simulink library "canBswLib"  (R2023b)
settings: Solver=VariableStepAuto  StartTime=0.0  StopTime=10.0  RelTol=1e-3
undefined symbols (not defined in the file): Data, Extended, ID, Length
libraries: can_bswapi x15, simulink x12, hdlsllib x5, $bdroot x4, dspswit3 x2, bamFsm x1
settings Model: Creator=zon07  LastModifiedBy=Professional
settings SFSimCC: SimTargetLang=C++

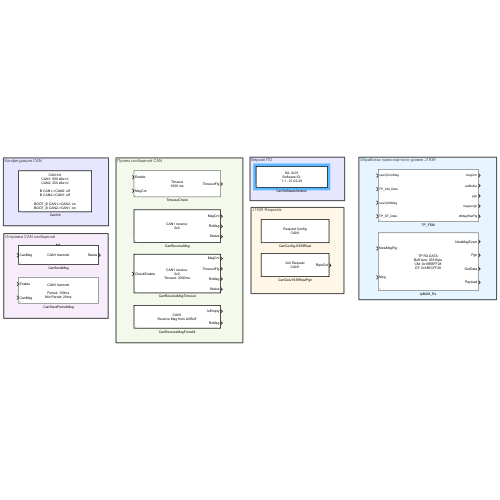
[thumbnail: Simulink's stored preview of the top-level diagram]
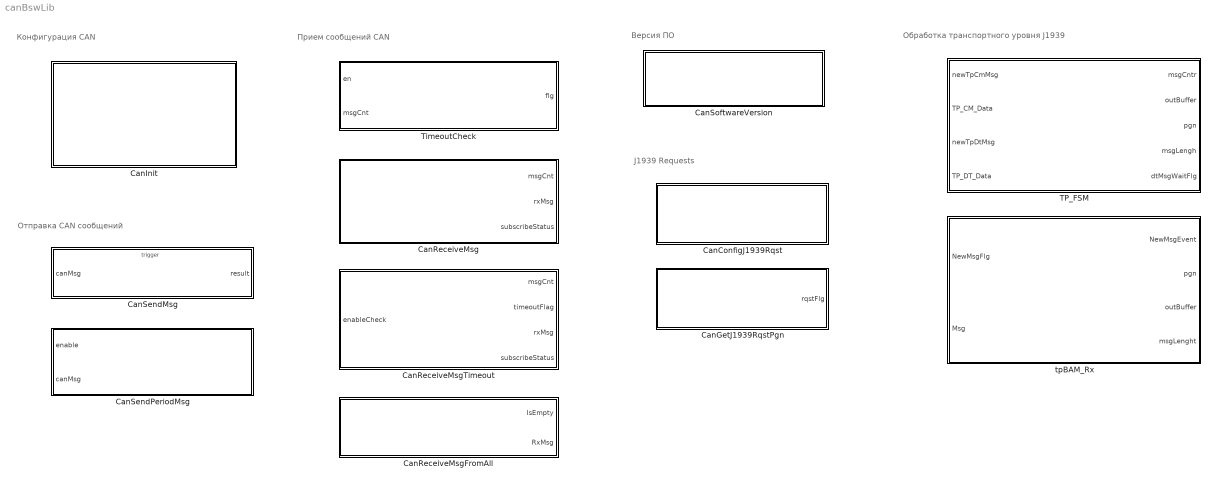
== system canBswLib ==
  note: Обработка транспортного уровня J1939
  note: Версия ПО
  note: J1939 Requests
  note: Отправка CAN сообщений
  note: Конфигурация CAN
  note: Прием сообщений CAN
  CanConfigJ1939Rqst : Subsystem  TreatAsAtomicUnit=on  mask(Request Config){can='CAN1', id=0x18EA3128, onlyPgnFlg=on, fromAllFlg=on}
      mask prompts: can "CAN Number"; id "Rqst Id:"; onlyPgnFlg "Принимать только по PGN"; fromAllFlg "Принимать запрос "Для всех""
      mask help:
      | Данный блок устанавливает с какого ID будут приниматься запросы.
      | CAN Number: номер CAN;
      | Rqst Id: Id запроса;
      | Флаг "Флаг принимать только по PGN" - SA источника запроса будет игнорироваться;
      | Флаг "Принимать запрос "Для всех" - Пример если установлен 0x18EA3128, так же будет обрабатываться 0x18EAFF28;
      mask init:
      | block_name = "Request Config\n" + "CAN" + num2str(can);
      mask TypeOptions can: 'CAN1' | 'CAN2'
      mask DialogControl ParameterGroupVar Prompt: CAN:
      mask DialogControl Container3 Prompt: Parameters
      mask Display: disp(block_name);
  CanGetJ1939RqstPgn : Subsystem  TreatAsAtomicUnit=on  mask(Get request for PGN){can='CAN1', pgn=0x0000}
      mask prompts: can "CAN Number"
      mask help:
      | Функция возвращает true на один шаг,если был получен запрос на утсановленный PGN.
      | Максимум 16 уникальных Pgn.
      mask init:
      | block_name = "0x" + dec2hex(pgn) + " Request\n" + "CAN" + num2str(can);
      mask TypeOptions can: 'CAN1' | 'CAN2'
      mask DialogControl ParameterGroupVar Prompt: CAN
      mask Display:
      | disp(block_name)
      | port_label('output', 1, 'RqstСnt');
  CanSoftwareVersion : Subsystem  LoadFcn=|  TreatAsAtomicUnit=on  mask(Software Version CAN){software_version=0, model_number=1, version=1, subversion=1, firmware_date="21.02.25", date_update=on, sa=0x31, id=0x18EAFF28, id_1=0x18EAFF28}
      | null_str = """00.00.00""";
      | read_str = get_param(gcb, 'firmware_date');
      | 
      | if (read_str == null_str)
      |     write_str = """" + string(datetime('now', 'Format', 'dd.MM.yy')) + """";
      |     set_param(gcb, 'firmware_date', write_str);
      | end
      | 
      | update = get_param(gcb, 'date_update');
      | 
      | switch (update)
      |     case 'on'
      |         write_str = """" + string(datetime('now', 'Format', 'dd.MM.yy')) + """";
      |         set_param(gcb, 'firmware_date', write_str);
      |     case 'off'
      |         %Nothing to do
      | end
      | 
      | clear null_str read_str write_str update;
      mask prompts: software_version "Software version"; model_number "Model number:"; version "Firmware version:"; subversion "Firmware subversion:"; firmware_date "Date:"; date_update "Update on model startup"; id "Message ID:"; id_1 "Message ID:"
      mask help: Процесс приема запроса и отправки версии ПО в CAN согласно J1939.
      mask init:
      | software_version = char(3) + "-" + num2str(model_number, '%02.0f') + "*" + num2str(version, '%02.0f') + "." + num2str(subversion) + "*" + firmware_date + "*";
      | block_name = "SA: 0x" + num2str(dec2hex(sa)) + "\nSoftware ID:\n" + num2str(version) + "." + num2str(subversion) + " - " + firmware_date;
      settings: CopyFcn=|
      | null_str = """00.00.00""";
      | read_str = get_param(gcb, 'firmware_date');
      | 
      | if (read_str == null_str)
      |     write_str = """" + string(datetime('now', 'Format', 'dd.MM.yy')) + """";
      |     set_param(gcb, 'firmware_date', write_str);
      | end
      | 
      | clear null_str read_str write_str;
      settings: MoveFcn=|
      | null_str = """00.00.00""";
      | read_str = get_param(gcb, 'firmware_date');
      | 
      | if (read_str == null_str)
      |     write_str = """" + string(datetime('now', 'Format', 'dd.MM.yy')) + """";
      |     set_param(gcb, 'firmware_date', write_str);
      | end
      | 
      | clear null_str read_str write_str;
      mask TypeOptions id: СanReceiveMsg/id
      mask TypeOptions id_1: СanReceiveMsg1/id
      mask DialogControl ParameterGroupVar Prompt: Firmware version
      mask DialogControl Container3 Prompt: Date
      mask DialogControl Container6 Prompt: CAN SA
      mask DialogControl Container4 Prompt: CAN1 Request
      mask DialogControl Container5 Prompt: CAN2 Request
      mask Display: disp(block_name);
  TP_FSM : Subsystem  mask(J1939 TP Msg Rx Fsm){buffSize=255}
      mask prompts: buffSize "Размер буффера, байт:"
      mask help: Машина состояний приема сообщений по Transport Protocol J1939
  TimeoutCheck : Subsystem  mask(Check TimeOut){timeout_ms=1000}
      mask prompts: timeout_ms "Timeout, ms"
      mask help: Проверка таймаута для CAN сообщений
      mask init:
      | block_name = "Timeout\n" + num2str(timeout_ms) + " ms";
      mask DialogControl ParameterGroupVar Prompt: Параметры
      mask Display:
      | disp(block_name);
      | port_label('input', 1, 'Enable');
      | port_label('input', 2, 'MsgCnt');
      | port_label('output', 1, 'TimeoutFlg');
  tpBAM_Rx : Subsystem  mask(TP RX DATA){tpCmId=0x18EBFF28, tpDtId=0x18ECFF28, buffSize=255}
      mask prompts: tpCmId "CAN ID TP.CM:"; tpDtId "CAN ID DT.CM:"; buffSize "Размер буффера, байт:"
      mask help:
      | Прием сообщений по транспортному протоколу J1939.
      | Порты:
      | 1) NewMsgEvent - событие(вызов) при получении(сборке) нового сообщения;
      | 2) Pgn - PGN принятого сообщений;
      | 3) OutData - массив данных собранного сообщений (длина равна BuffSize заданного в настройках);
      | 4) MsgLenght - длина полезных данных в буффере;
      | 5) DtMsgWaitFlg - флаг ожидания приема сообщения данных TP.DT;
      |
      | !!! При неудачном приеме - буффер очищается (0xFF).
      mask init:
      | blockName = "TP RX DATA\n" + "Buff size: " + num2str(buffSize) + " Byte"...
      |                 + "\nCM: 0x" + dec2hex(tpCmId)...
      |                 + "\nDT: 0x" + dec2hex(tpDtId);
      mask TypeOptions buffSize: TP_FSM/buffSize
      mask DialogControl ParameterGroupVar Prompt: Параметры
      mask Display:
      | disp(blockName);
      | port_label('input', 1, 'NewMsgFlg');
      | port_label('input', 2, 'Msg');
      | 
      | port_label('output', 1, 'NewMsgEvent');
      | port_label('output', 3, 'OutData');
      | port_label('output', 2, 'Pgn');
      | port_label('output', 4, 'Payload');
  СanInit : Subsystem  TreatAsAtomicUnit=on  mask(Инициализация CAN){bitrate_can_1=500 кбит/с, brigdeCan1to2Flg=off, bootBrigdeCan1to2Flg=on, bitrate_can_2=250 кбит/с, brigdeCan2to1Flg=off, bootBrigdeCan2to1Flg=on}
      mask prompts: bitrate_can_1 "Скорость шины CAN 1"; brigdeCan1to2Flg "Проброс сообщений из CAN1 в CAN2"; bootBrigdeCan1to2Flg "Проброс сообщений бутлоадера из CAN1 в CAN2"; bitrate_can_2 "Скорость шины CAN 2"; brigdeCan2to1Flg "Проброс сообщений из CAN2 в CAN1"; bootBrigdeCan2to1Flg "Проброс сообщений бутлоадера из CAN2 в CAN1"
      mask help:
      | Выбор скорости передачи данных для CAN1 и CAN2;
      | Выбор необходимости Bridge-режима (проброса) для каждого CAN;
      | BOOT_RS_ID - CAN_ID по которому будет происходить сброс контроллера (возможно уберем в будущем).
      mask init:
      | maskObj = Simulink.Mask.get(gcb);
      | speedCan1 = maskObj.getParameter('bitrate_can_1').Value;
      | speedCan2 = maskObj.getParameter('bitrate_can_2').Value;
      | 
      | bridge1_2 = maskObj.getParameter('brigdeCan1to2Flg').Value;
      | bridge2_1 = maskObj.getParameter('brigdeCan2to1Flg').Value;
      | 
      | bootBrigde1_2 = maskObj.getParameter('bootBrigdeCan1to2Flg').Value;
      | bootBrigde2_1 = maskObj.getParameter('bootBrigdeCan2to1Flg').Value;
      | 
      | block_name = "CAN Init" + "\n" + "CAN1: " + speedCan1...
      |                         + "\n" + "CAN2: " + speedCan2...
      |                         + "\n\n" + "B CAN1->CAN2: " + bridge1_2...
      |                         + "\n" + "B CAN2->CAN1: " + bridge2_1...
      |                         + "\n\n" + "BOOT_B CAN1->CAN2: " + bootBrigde1_2...
      |                         + "\n" + "BOOT_B CAN2->CAN1: " + bootBrigde2_1;
      mask TypeOptions bitrate_can_1: 125 кбит/с | 250 кбит/с | 500 кбит/с | 1000 кбит/с
      mask TypeOptions bitrate_can_2: 125 кбит/с | 250 кбит/с | 500 кбит/с | 1000 кбит/с
      mask DialogControl Container Prompt: CAN1
      mask DialogControl Container1 Prompt: CAN2
      mask Display: disp(block_name);
  СanReceiveMsg : Subsystem  TreatAsAtomicUnit=on  mask(Прием Can-сообщения по "подписке"){can=CAN1, id=0x0, sample_time=-1}
      mask prompts: id "Message ID:"; sample_time "Sample time:"
      mask help:
      | Задайте идентификатор сообщения CAN которое необходимо получать.
      |
      | На выходе rxMsg данные будут в виде BUS:CAN_MESSAGE_BUS
      | На выходе msgCnt будет счетчик количества принятых собщений uint32.
      |
      | Ограничение на количество блоков с уникальным ID - 128 блока (с учетом СanReceiveMsgTimeout) для кажого модуля CAN.
      | Если количество ID превышено и подписка не удалась, на выходе Status будет значение False (0) ;
      |
      | Sample time - период выполнения блока. Должен быть больше шага моделирования. Значение -1 задаёт Sample time как наследуемый.
      mask init:
      | block_name = "CAN" + num2str(can) + " receive:\n0x" + dec2hex(id);
      mask TypeOptions can: CAN1 | CAN2
      mask DialogControl ParameterGroupVar Prompt: Параметры
      mask Display:
      | disp(block_name);
      | port_label('output', 1, 'MsgCnt');
      | port_label('output', 2, 'RxMsg');
      | port_label('output', 3, 'Status');
  СanReceiveMsgFromAll : Subsystem  TreatAsAtomicUnit=on  mask(Получить сообщений из кольцевого буффера CAN){can=CAN1}
      mask help:
      | Получение сообщения из кольцевого буффера CAN.
      | IsEmpty - Флаг сигнализирующий, что буффер пуст.
      |
      | Одиночный вызов - считает одно сообщение из буффера.
      | Данный блок целесообразно использовать в конструкции с циклом while.
      | Так можно считывать все сообщения(и повторяющиеся ID) принятые за шаг выполнения.
      mask init:
      | block_name = "CAN" + num2str(can) + "\nReceive Msg from All Buff";
      mask TypeOptions can: CAN1 | CAN2
      mask DialogControl ParameterGroupVar Prompt: Параметры
      mask Display:
      | disp(block_name);
      | port_label('output', 1, 'IsEmpty');
      | port_label('output', 2, 'RxMsg');
  СanReceiveMsgTimeout : Subsystem  TreatAsAtomicUnit=on  mask(Can Message Rx){id=0, can='CAN1', timeout_ms=2000, sample_time=-1}
      mask prompts: timeout_ms "Timeout, ms"; sample_time "Sample time, s:"
      mask help:
      | Задайте идентификатор сообщения CAN которое необходимо получать.
      |
      | На выходе rxMsg данные будут в виде BUS:CAN_MESSAGE_BUS
      | На выходе msgCnt будет счетчик количества принятых собщений uint32.
      |
      | Ограничение на количество блоков с уникальным ID - 128 блока(с учетом СanReceiveMsg)для кажого модуля CAN.
      | Если количество ID превышено и подписка не удалась, на выходе Status будет значение False (0) ;
      |
      | Sample time - период выполнения блока. Должен быть больше шага моделирования. Значение -1 задаёт Sample time как наследуемый.
      |
      | enableCheck - включение контроля таймаута;
      | timeoutFlg - флаг контроля таймаута сообщения;
      mask init:
      | block_name = "CAN" + num2str(can) + " receive:\n0x" + dec2hex(id) + "\nTimeout: " + timeout_ms + "ms";
      mask TypeOptions can: 'CAN1' | 'CAN2'
      mask DialogControl Container2 Prompt: Параметры
      mask Display:
      | disp(block_name);
      | port_label('output', 1, 'MsgCnt');
      | port_label('output', 2, 'TimeoutFlg');
      | port_label('output', 3, 'RxMsg');
      | port_label('output', 4, 'Status');
      | port_label('input', 1, 'CheckEnable');
  СanSendMsg : Subsystem  mask(Отправка сообщения CAN){can=CAN1}
      mask help:
      | Выберите CAN шину для передачи сообщения.
      |
      | Порт canMsg - Сообщение для отправки типа Bus: CAN_MESSAGE_BUS.
      |
      | Данный блок, при вызове, поместит сообщений в очередь CAN для отправки.
      |
      | Status - статус выполнения функции (Тип Enum: Statuses)
      mask init:
      | blockName = "CAN" + num2str(can) + " transmit";
      mask TypeOptions can: CAN1 | CAN2
      mask DialogControl ParameterGroupVar Prompt: Параметры
      mask Display:
      | disp(blockName);
      | port_label('input', 1, 'CanMsg');
      | port_label('output', 1, 'Status');
  СanSendPeriodMsg : Subsystem  mask(CanSend){by_period=on, by_dataChange=off, can=CAN1, period_time=0.1, sample_time=0.02}
      mask prompts: by_period "Периодическая отправка"; by_dataChange "По изменению данных"; period_time "Период , сек:"; sample_time "Минимальный период, сек:"
      mask help: Выберите CAN шину для передачи сообщения.<br>Sample time - период выполнения блока. Должен быть больше шага моделирования. Значение -1 задаёт Sample time как наследуемый.<br><br>-Порт enable - включения/выключения отправки.<br>-Порт canMsg - Сообщение для отправки типа Bus: CAN_MESSAGE_BUS(можно создать коммандой canMessageBusType, скопировать и поместить в словарь модели)
      mask init:
      | block_name = "CAN" + num2str(can) + " transmit";
      | period = num2str(period_time * 1000)+ "ms";
      | 
      | if(sample_time == -1)
      |     min_period = "Inherit";
      | else
      |     min_period = num2str(sample_time * 1000)+ "ms";  
      | end
      | 
      | if(by_period == true && by_dataChange == false)
      |     block_name = "CAN" + num2str(can) + " transmit\n\n" + "Period: " + period + "\nMin Period: " + min_period;
      | elseif(by_period == true && by_dataChange == true)
      |     block_name = "CAN" + num2str(can) + " transmit\n\n" + "By Data Change\n" + "Period: " + period + "\nMin Period: " + min_period;
      | elseif(by_period == false && by_dataChange == true)
      |     block_name = "CAN" + num2str(can) + " transmit\n\n" + "By Data Change" + "\nMin Period: " + min_period;
      | else
      |     block_name = "CAN" + num2str(can) + " transmit OFF";
      | end
      mask TypeOptions can: CAN1 | CAN2
      mask DialogControl Container4 Prompt: Настройки:
      mask DialogControl ParameterGroupVar Prompt: Параметры
      mask DialogControl Container3 Prompt: Периоды
      mask Display:
      | disp(block_name);
      | port_label('input', 1, 'Enable');
      | port_label('input', 2, 'CanMsg');

== system canBswLib/CanConfigJ1939Rqst ==
  Constant1 : Constant  Value=0
  Initialize Function : Subsystem  TreatAsAtomicUnit=on
  Terminator : Terminator
  wires:
  Constant1/1 -> Terminator/1

== system canBswLib/CanGetJ1939RqstPgn ==
  Constant : Constant  Value=pgn  OutDataTypeStr=uint32
  Initialize Function : Subsystem  TreatAsAtomicUnit=on
  can : Constant  Value=(can - 1)  OutDataTypeStr=int32
  canApi_getRqstJ1939 : can_bswapi/canApi_getRqstJ1939  SampleTime=-1
  rqstFlg : Outport  OutDataTypeStr=uint32
  wires:
  Constant/1 -> canApi_getRqstJ1939/2
  canApi_getRqstJ1939/1 -> rqstFlg/1
  can/1 -> canApi_getRqstJ1939/1

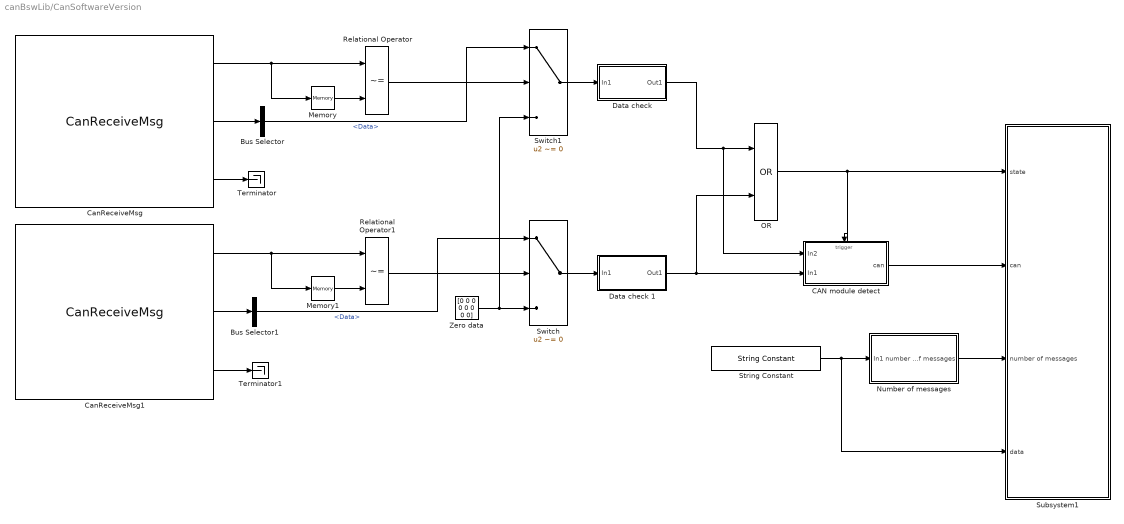
== system canBswLib/CanSoftwareVersion ==
  Bus Selector : BusSelector  OutputSignals=Data
  Bus Selector1 : BusSelector  OutputSignals=Data
  CAN module detect : Subsystem  TreatAsAtomicUnit=on
  Data check : Subsystem
  Data check 1 : Subsystem
  Memory : Memory
  Memory1 : Memory
  Number of messages : Subsystem
  OR : Logic  Operator=OR  AllPortsSameDT=off  OutDataTypeStr=boolean
  Relational Operator : RelationalOperator  Operator=~=  OutDataTypeStr=boolean  RndMeth=Simplest  InputSameDT=off
  Relational Operator1 : RelationalOperator  Operator=~=  OutDataTypeStr=boolean  RndMeth=Simplest  InputSameDT=off
  String Constant : StringConstant  String=software_version
  Subsystem1 : Subsystem
  Switch : Switch  Criteria=u2 ~= 0  RndMeth=Simplest  SaturateOnIntegerOverflow=off  InputSameDT=off
  Switch1 : Switch  Criteria=u2 ~= 0  RndMeth=Simplest  SaturateOnIntegerOverflow=off  InputSameDT=off
  Terminator : Terminator
  Terminator1 : Terminator
  Zero data : Constant  Value=[0 0 0 0 0 0 0 0]  OutDataTypeStr=uint8
  СanReceiveMsg : $bdroot/СanReceiveMsg  can=CAN1  id=id  sample_time=0.2
  СanReceiveMsg1 : $bdroot/СanReceiveMsg  can=CAN2  id=id_1  sample_time=0.2
  wires:
  СanReceiveMsg/3 -> Terminator/1
  СanReceiveMsg1/3 -> Terminator1/1
  Bus Selector1/1 -> Switch/1  "<Data>"
  Relational Operator1/1 -> Switch/2
  Memory1/1 -> Relational Operator1/2
  СanReceiveMsg1/1 -> Relational Operator1/1, Memory1/1
  СanReceiveMsg1/2 -> Bus Selector1/1
  Bus Selector/1 -> Switch1/1  "<Data>"
  СanReceiveMsg/2 -> Bus Selector/1
  Relational Operator/1 -> Switch1/2
  СanReceiveMsg/1 -> Relational Operator/1, Memory/1
  Memory/1 -> Relational Operator/2
  CAN module detect/1(can) -> Subsystem1/2(can)
  OR/1 -> Subsystem1/1(state), CAN module detect/Trigger
  Data check 1/1(Out1) -> CAN module detect/2(In1), OR/2
  Data check/1(Out1) -> CAN module detect/1(In2), OR/1
  Switch/1 -> Data check 1/1(In1)
  Switch1/1 -> Data check/1(In1)
  Zero data/1 -> Switch/3, Switch1/3
  String Constant/1 -> Number of messages/1(In1), Subsystem1/4(data)
  Number of messages/1(number of messages) -> Subsystem1/3(number of messages)

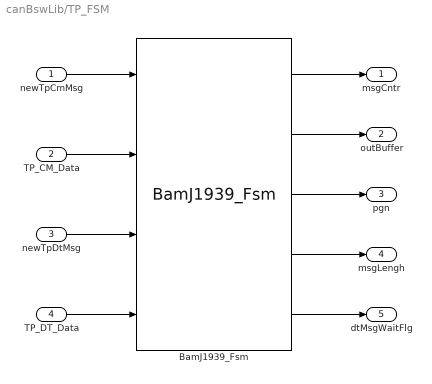
== system canBswLib/TP_FSM ==
  newTpCmMsg : Inport
  TP_CM_Data : Inport  Port=2
  newTpDtMsg : Inport  Port=3
  TP_DT_Data : Inport  Port=4
  BamJ1939_Fsm : bamFsm/BamJ1939_Fsm  SystemSampleTime=-1  VariantActivationTime=update diagram  AllowFlexibleInterface=on  Latency=0  AutoFrameSizeCalculation=off
      settings: PortSchema="{\"entries\":[{\"content\":{\"sides\":[{\"content\":{\"connectorIds\":[\"In3\",\"In1\",\"In4\",\"In2\"]},\"type\":\"ConnectorPlacement.EquallySpacedRectSide\",\"uuid\":\"f0437618-7372-46d8-9ab7-ff8929e6fb67\"},{\"content\":{\"connectorIds\":[\"Out2\",\"Out1\",\"Out3\",\"Out4\",\"Out5\"],\"side\":\"RIGHT\"},\"type\":\"ConnectorPlacement.EquallySpacedRectSide\",\"uuid\":\"0536630b-4cc4-4e97-9664-ff8fdcddfe97\"},{\"content\":{\"side\":\"TOP\"},\"type\":\"ConnectorPlacement.EquallySpacedRectSide\",\"uuid\":\"62369740-83f5-4f7d-ae2b-bf987bd5a7ae\"}]},\"type\":\"ConnectorPlacement.EquallySpacedConnector\",\"uuid\":\"7025f99e-73e8-416b-8734-672140f8b319\"}],\"packageUris\":[\"http://schema.mathworks.com/mf0/Connector/R2020b\"],\"version\":\"1.0\"}"
  msgCntr : Outport
  outBuffer : Outport  Port=2
  pgn : Outport  Port=3
  msgLengh : Outport  Port=4
  dtMsgWaitFlg : Outport  Port=5  OutDataTypeStr=boolean
  wires:
  BamJ1939_Fsm/5 -> dtMsgWaitFlg/1
  BamJ1939_Fsm/4 -> msgLengh/1
  BamJ1939_Fsm/2 -> msgCntr/1
  BamJ1939_Fsm/3 -> pgn/1
  BamJ1939_Fsm/1 -> outBuffer/1
  TP_CM_Data/1 -> BamJ1939_Fsm/1
  newTpCmMsg/1 -> BamJ1939_Fsm/3
  newTpDtMsg/1 -> BamJ1939_Fsm/4
  TP_DT_Data/1 -> BamJ1939_Fsm/2

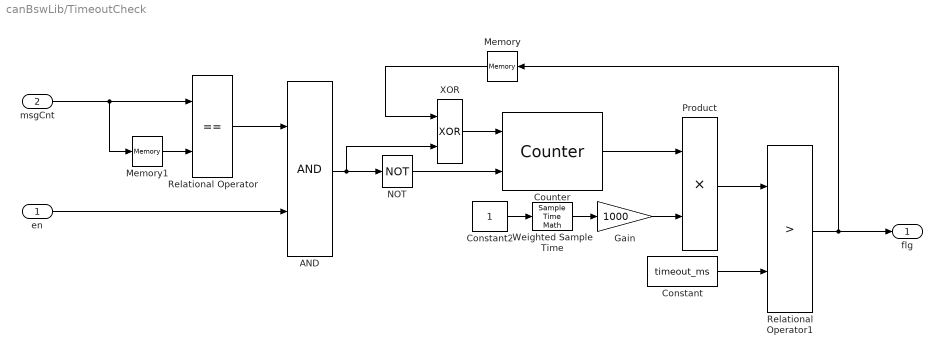
== system canBswLib/TimeoutCheck ==
  en : Inport
  msgCnt : Inport  Port=2
  AND : Logic  AllPortsSameDT=off  OutDataTypeStr=boolean
  Constant : Constant  Value=timeout_ms  OutDataTypeStr=uint32
  Constant2 : Constant  OutDataTypeStr=uint32
  Counter : dspswit3/Counter  Direction=Up  CountEvent=Non-zero sample  CounterSize=16 bits  MaxCount=255  InitialCount=0  Output=Count  HitValue=32  ResetInput=on  SamplesPerFrame=1  Ts=-1  CntDtype=uint16  HitDtype=Logical
  Gain : Gain  Gain=1000  ParamDataTypeStr=single  OutDataTypeStr=uint32  RndMeth=Simplest
  Memory : Memory  InheritSampleTime=on
  Memory1 : Memory  InheritSampleTime=on
  NOT : Logic  Operator=NOT  IconShape=distinctive  AllPortsSameDT=off  OutDataTypeStr=boolean
  Product : Product  OutDataTypeStr=uint32  RndMeth=Simplest
  Relational Operator : RelationalOperator  Operator===  OutDataTypeStr=boolean  ZeroCross=off  RndMeth=Simplest  InputSameDT=off
  Relational Operator1 : RelationalOperator  Operator=>  OutDataTypeStr=boolean  ZeroCross=off  RndMeth=Simplest  InputSameDT=off
  Weighted Sample Time : SampleTimeMath  TsampMathOp=Ts Only  weightValue=uint32(1)  OutDataTypeStr=single
  XOR : Logic  Operator=XOR  AllPortsSameDT=off  OutDataTypeStr=boolean
  flg : Outport
  wires:
  Memory1/1 -> Relational Operator/2
  AND/1 -> XOR/2, NOT/1
  msgCnt/1 -> Memory1/1, Relational Operator/1
  Relational Operator/1 -> AND/1
  Relational Operator1/1 -> Memory/1, flg/1
  en/1 -> AND/2
  Constant/1 -> Relational Operator1/2
  Constant2/1 -> Weighted Sample Time/1
  Weighted Sample Time/1 -> Gain/1
  Product/1 -> Relational Operator1/1
  Counter/1 -> Product/1
  Gain/1 -> Product/2
  NOT/1 -> Counter/2
  XOR/1 -> Counter/1
  Memory/1 -> XOR/1

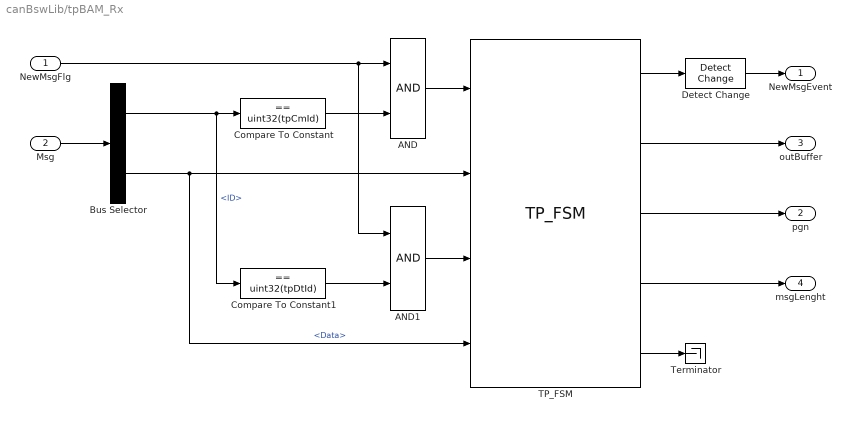
== system canBswLib/tpBAM_Rx ==
  NewMsgFlg : Inport  OutDataTypeStr=boolean
  Msg : Inport  Port=2  OutDataTypeStr=Bus: CAN_MESSAGE_BUS
  AND : Logic  AllPortsSameDT=off  OutDataTypeStr=boolean
  AND1 : Logic  AllPortsSameDT=off  OutDataTypeStr=boolean
  Bus Selector : BusSelector  OutputSignals=ID,Data
  Compare To Constant : simulink/Logic and Bit Operations/Compare To Constant  relop===  const=uint32(tpCmId)  OutDataTypeStr=boolean  ZeroCross=off
  Compare To Constant1 : simulink/Logic and Bit Operations/Compare To Constant  relop===  const=uint32(tpDtId)  OutDataTypeStr=boolean  ZeroCross=off
  Detect Change : simulink/Logic and Bit Operations/Detect Change  vinit=0  OutDataTypeStr=boolean
  TP_FSM : $bdroot/TP_FSM  buffSize=buffSize
  Terminator : Terminator
  NewMsgEvent : Outport
  pgn : Outport  Port=2
  outBuffer : Outport  Port=3
  msgLenght : Outport  Port=4
  wires:
  TP_FSM/5 -> Terminator/1
  Msg/1 -> Bus Selector/1
  Compare To Constant1/1 -> AND1/2
  AND1/1 -> TP_FSM/3
  NewMsgFlg/1 -> AND/1, AND1/1
  Compare To Constant/1 -> AND/2
  AND/1 -> TP_FSM/1
  Bus Selector/2 -> TP_FSM/4, TP_FSM/2  "<Data>"
  Bus Selector/1 -> Compare To Constant/1, Compare To Constant1/1  "<ID>"
  TP_FSM/2 -> outBuffer/1
  TP_FSM/3 -> pgn/1
  TP_FSM/4 -> msgLenght/1
  Detect Change/1 -> NewMsgEvent/1
  TP_FSM/1 -> Detect Change/1

== system canBswLib/СanInit ==
  Function-Call Generator : simulink/Ports & Subsystems/Function-Call Generator  sample_time=-1  numberOfIterations=1  DisallowWideOutput=off
  Function-Call Subsystem : Subsystem  TreatAsAtomicUnit=on
  Initialize Function : Subsystem  TreatAsAtomicUnit=on
  wires:
  Function-Call Generator/1 -> Function-Call Subsystem/Trigger

== system canBswLib/СanReceiveMsg ==
  Bus Assignment : BusAssignment  AssignedSignals=Extended,ID,Length,Data
  Bus Selector : BusSelector  OutputSignals=id,length,data
  CAN Receive : Subsystem  TreatAsAtomicUnit=on
  Function-Call Generator : simulink/Ports & Subsystems/Function-Call Generator  sample_time=sample_time  numberOfIterations=1  DisallowWideOutput=off
  Initialize Function : Subsystem  TreatAsAtomicUnit=on
  initCanBus : Constant  Value=0  OutDataTypeStr=Bus: CAN_MESSAGE_BUS
  initExtd : Constant  OutDataTypeStr=uint8
  msgCnt : Outport
  rxMsg : Outport  Port=2  OutDataTypeStr=Bus: CAN_MESSAGE_BUS
  subscribeStatus : Outport  Port=3
  wires:
  Bus Selector/1 -> Bus Assignment/3  "<id>"
  Bus Selector/3 -> Bus Assignment/5  "<data>"
  Bus Selector/2 -> Bus Assignment/4  "<length>"
  CAN Receive/2(rxMsg) -> Bus Selector/1
  Initialize Function/1(subscribeStatus) -> subscribeStatus/1
  initExtd/1 -> Bus Assignment/2
  Bus Assignment/1 -> rxMsg/1
  initCanBus/1 -> Bus Assignment/1
  CAN Receive/1(msgCnt) -> msgCnt/1
  Function-Call Generator/1 -> CAN Receive/Trigger

== system canBswLib/СanReceiveMsgFromAll ==
  Bus Assignment : BusAssignment  AssignedSignals=Extended,ID,Length,Data
  Bus Selector : BusSelector  OutputSignals=id,length,data
  can : Constant  Value=(can - 1)  OutDataTypeStr=int32
  canApi_GetAllMessages : can_bswapi/canApi_GetAllMessages  SampleTime=-1
  initCanBus : Constant  Value=0  OutDataTypeStr=Bus: CAN_MESSAGE_BUS
  initExtd : Constant  OutDataTypeStr=uint8
  IsEmpty : Outport
  RxMsg : Outport  Port=2  OutDataTypeStr=Bus: CAN_MESSAGE_BUS
  wires:
  Bus Assignment/1 -> RxMsg/1
  initCanBus/1 -> Bus Assignment/1
  Bus Selector/2 -> Bus Assignment/4  "<length>"
  canApi_GetAllMessages/2 -> Bus Selector/1
  initExtd/1 -> Bus Assignment/2
  Bus Selector/3 -> Bus Assignment/5  "<data>"
  Bus Selector/1 -> Bus Assignment/3  "<id>"
  canApi_GetAllMessages/1 -> IsEmpty/1
  can/1 -> canApi_GetAllMessages/1

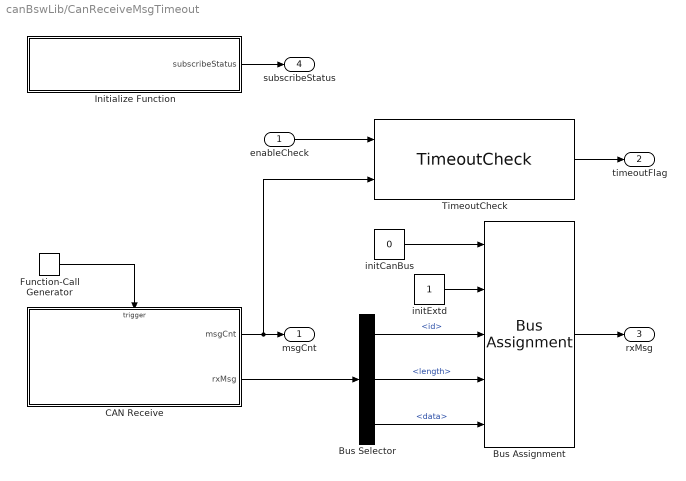
== system canBswLib/СanReceiveMsgTimeout ==
  enableCheck : Inport  OutDataTypeStr=boolean
  Bus Assignment : BusAssignment  AssignedSignals=Extended,ID,Length,Data
  Bus Selector : BusSelector  OutputSignals=id,length,data
  CAN Receive : Subsystem  TreatAsAtomicUnit=on
  Function-Call Generator : simulink/Ports & Subsystems/Function-Call Generator  sample_time=sample_time  numberOfIterations=1  DisallowWideOutput=off
  Initialize Function : Subsystem  TreatAsAtomicUnit=on
  TimeoutCheck : $bdroot/TimeoutCheck  timeout_ms=timeout_ms
  initCanBus : Constant  Value=0  OutDataTypeStr=Bus: CAN_MESSAGE_BUS
  initExtd : Constant  OutDataTypeStr=uint8
  msgCnt : Outport
  timeoutFlag : Outport  Port=2
  rxMsg : Outport  Port=3  OutDataTypeStr=Bus: CAN_MESSAGE_BUS
  subscribeStatus : Outport  Port=4
  wires:
  Bus Selector/3 -> Bus Assignment/5  "<data>"
  Bus Selector/1 -> Bus Assignment/3  "<id>"
  CAN Receive/2(rxMsg) -> Bus Selector/1
  Initialize Function/1(subscribeStatus) -> subscribeStatus/1
  TimeoutCheck/1 -> timeoutFlag/1
  enableCheck/1 -> TimeoutCheck/1
  CAN Receive/1(msgCnt) -> TimeoutCheck/2, msgCnt/1
  initExtd/1 -> Bus Assignment/2
  initCanBus/1 -> Bus Assignment/1
  Bus Assignment/1 -> rxMsg/1
  Bus Selector/2 -> Bus Assignment/4  "<length>"
  Function-Call Generator/1 -> CAN Receive/Trigger

== system canBswLib/СanSendMsg ==
  canMsg : Inport  OutDataTypeStr=Bus: CAN_MESSAGE_BUS
  function : TriggerPort  TriggerType=function-call  VariantControl=(inherit)
  Bus Selector : BusSelector  OutputSignals=ID,Length,Data
  Cast : DataTypeConversion  OutDataTypeStr=Enum: Statuses  RndMeth=Simplest  SaturateOnIntegerOverflow=off
  can : Constant  Value=(can - 1)  OutDataTypeStr=int32
  canApi_SendMessage : can_bswapi/canApi_SendMessage  SampleTime=-1
  result : Outport  OutDataTypeStr=Enum: Statuses
  wires:
  canMsg/1 -> Bus Selector/1
  can/1 -> canApi_SendMessage/1
  canApi_SendMessage/1 -> Cast/1
  Bus Selector/1 -> canApi_SendMessage/2  "<ID>"
  Bus Selector/2 -> canApi_SendMessage/3  "<Length>"
  Bus Selector/3 -> canApi_SendMessage/4  "<Data>"
  Cast/1 -> result/1

== system canBswLib/СanSendPeriodMsg ==
  enable : Inport  OutDataTypeStr=boolean
  canMsg : Inport  Port=2  OutDataTypeStr=Bus: CAN_MESSAGE_BUS
  CanTxPMsg : Subsystem  TreatAsAtomicUnit=on  SystemSampleTime=sample_time
  wires:
  canMsg/1 -> CanTxPMsg/2(data)
  enable/1 -> CanTxPMsg/1(enable)

== system canBswLib/CanConfigJ1939Rqst/Initialize Function ==
  Constant : Constant  Value=id  OutDataTypeStr=uint32
  Constant1 : Constant  Value=onlyPgnFlg  OutDataTypeStr=boolean
  Constant2 : Constant  Value=fromAllFlg  OutDataTypeStr=boolean
  Event Listener : EventListener  DisableCoverage=on  EventName=reset
  can : Constant  Value=(can - 1)  OutDataTypeStr=int32
  canApi_confiqRqstId : can_bswapi/canApi_confiqRqstId  SampleTime=-1
  wires:
  Constant2/1 -> canApi_confiqRqstId/4
  Constant1/1 -> canApi_confiqRqstId/3
  Constant/1 -> canApi_confiqRqstId/2
  can/1 -> canApi_confiqRqstId/1

== system canBswLib/CanGetJ1939RqstPgn/Initialize Function ==
  Constant : Constant  Value=pgn  OutDataTypeStr=uint32
  Event Listener : EventListener  DisableCoverage=on  EventName=reset
  can : Constant  Value=(can - 1)  OutDataTypeStr=int32
  rqstSubscribe : can_bswapi/canApi_rqstSubscribe  SampleTime=-1
  wires:
  can/1 -> rqstSubscribe/1
  Constant/1 -> rqstSubscribe/2

== system canBswLib/CanSoftwareVersion/CAN module detect ==
  In2 : Inport
  In1 : Inport  Port=2
  Trigger : TriggerPort  VariantControl=(inherit)
  Cast : DataTypeConversion  OutDataTypeStr=int32  RndMeth=Simplest  SaturateOnIntegerOverflow=off
  Relational Operator : RelationalOperator  Operator=>  OutDataTypeStr=boolean  ZeroCross=off  RndMeth=Simplest  InputSameDT=off
  can : Outport
  wires:
  Cast/1 -> can/1
  Relational Operator/1 -> Cast/1
  In2/1 -> Relational Operator/2
  In1/1 -> Relational Operator/1

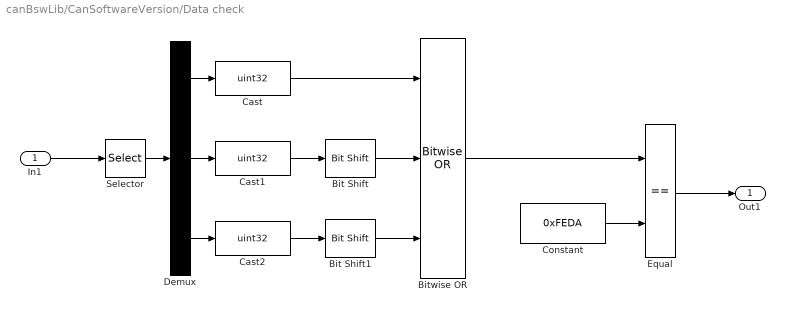
== system canBswLib/CanSoftwareVersion/Data check ==
  In1 : Inport
  Bit Shift : hdlsllib/Logic and Bit Operations/Bit Shift  mode=Shift Left Logical  N=8
  Bit Shift1 : hdlsllib/Logic and Bit Operations/Bit Shift  mode=Shift Left Logical  N=16
  Bitwise OR : simulink/Logic and Bit Operations/Bitwise Operator  logicop=OR  UseBitMask=off  NumInputPorts=3  BitMask=bin2dec('11011001')  BitMaskRealWorld=Stored Integer
      settings: LibrarySourceBlock=|
      | simulink/Quick Insert/Logic and Bit
      | Operations/Bitwise OR
  Cast : DataTypeConversion  OutDataTypeStr=uint32  ConvertRealWorld=Stored Integer (SI)  RndMeth=Simplest  SaturateOnIntegerOverflow=off
  Cast1 : DataTypeConversion  OutDataTypeStr=uint32  ConvertRealWorld=Stored Integer (SI)  RndMeth=Simplest  SaturateOnIntegerOverflow=off
  Cast2 : DataTypeConversion  OutDataTypeStr=uint32  ConvertRealWorld=Stored Integer (SI)  RndMeth=Simplest  SaturateOnIntegerOverflow=off
  Constant : Constant  Value=0xFEDA  OutDataTypeStr=uint32
  Demux : Demux  Outputs=3
  Equal : RelationalOperator  Operator===  OutDataTypeStr=boolean  RndMeth=Simplest  InputSameDT=off
  Selector : Selector  IndexMode=Zero-based  InputPortWidth=8  IndexOptions=Index vector (dialog)  Indices=[0 1 2]  OutputSizes=1
  Out1 : Outport
  wires:
  Bit Shift1/1 -> Bitwise OR/3
  Bit Shift/1 -> Bitwise OR/2
  Cast/1 -> Bitwise OR/1
  Bitwise OR/1 -> Equal/1
  Cast2/1 -> Bit Shift1/1
  Cast1/1 -> Bit Shift/1
  Demux/3 -> Cast2/1
  Demux/2 -> Cast1/1
  Demux/1 -> Cast/1
  Selector/1 -> Demux/1
  Equal/1 -> Out1/1
  In1/1 -> Selector/1
  Constant/1 -> Equal/2

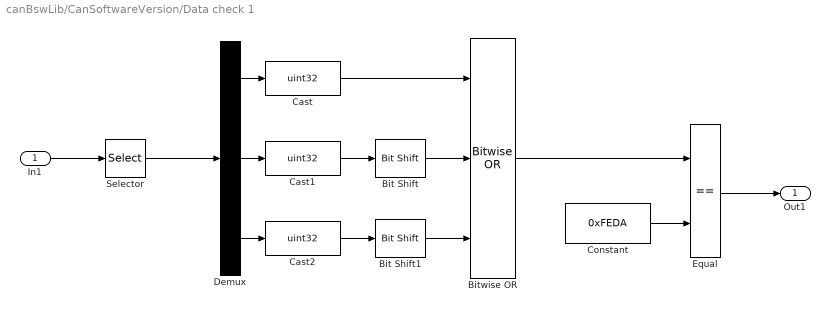
== system canBswLib/CanSoftwareVersion/Data check 1 ==
  In1 : Inport
  Bit Shift : hdlsllib/Logic and Bit Operations/Bit Shift  mode=Shift Left Logical  N=8
  Bit Shift1 : hdlsllib/Logic and Bit Operations/Bit Shift  mode=Shift Left Logical  N=16
  Bitwise OR : simulink/Logic and Bit Operations/Bitwise Operator  logicop=OR  UseBitMask=off  NumInputPorts=3  BitMask=bin2dec('11011001')  BitMaskRealWorld=Stored Integer
      settings: LibrarySourceBlock=|
      | simulink/Quick Insert/Logic and Bit
      | Operations/Bitwise OR
  Cast : DataTypeConversion  OutDataTypeStr=uint32  ConvertRealWorld=Stored Integer (SI)  RndMeth=Simplest  SaturateOnIntegerOverflow=off
  Cast1 : DataTypeConversion  OutDataTypeStr=uint32  ConvertRealWorld=Stored Integer (SI)  RndMeth=Simplest  SaturateOnIntegerOverflow=off
  Cast2 : DataTypeConversion  OutDataTypeStr=uint32  ConvertRealWorld=Stored Integer (SI)  RndMeth=Simplest  SaturateOnIntegerOverflow=off
  Constant : Constant  Value=0xFEDA  OutDataTypeStr=uint32
  Demux : Demux  Outputs=3
  Equal : RelationalOperator  Operator===  OutDataTypeStr=boolean  RndMeth=Simplest  InputSameDT=off
  Selector : Selector  IndexMode=Zero-based  InputPortWidth=8  IndexOptions=Index vector (dialog)  Indices=[0 1 2]  OutputSizes=1
  Out1 : Outport
  wires:
  Selector/1 -> Demux/1
  Demux/2 -> Cast1/1
  Demux/3 -> Cast2/1
  Bit Shift/1 -> Bitwise OR/2
  Cast2/1 -> Bit Shift1/1
  Bit Shift1/1 -> Bitwise OR/3
  Cast1/1 -> Bit Shift/1
  Bitwise OR/1 -> Equal/1
  Demux/1 -> Cast/1
  Cast/1 -> Bitwise OR/1
  Equal/1 -> Out1/1
  Constant/1 -> Equal/2
  In1/1 -> Selector/1

== system canBswLib/CanSoftwareVersion/Number of messages ==
  note: Количество посылок транспортным протоколом j1939
  In1 : Inport
  Add : Sum  OutDataTypeStr=uint8  RndMeth=Simplest
  Cast : DataTypeConversion  OutDataTypeStr=uint8  RndMeth=Simplest  SaturateOnIntegerOverflow=off
  Compare To Zero : simulink/Logic and Bit Operations/Compare To Zero  relop=~=  OutDataTypeStr=boolean
  Constant : Constant  Value=7  OutDataTypeStr=uint8
  Divide : Product  Inputs=*/  OutDataTypeStr=uint8  RndMeth=Simplest
  Mod : Math  Operator=mod
  String Length : StringLength  OutDataTypeStr=uint8
  number of messages : Outport
  wires:
  String Length/1 -> Divide/1, Mod/1
  Add/1 -> number of messages/1
  Compare To Zero/1 -> Cast/1
  In1/1 -> String Length/1
  Constant/1 -> Mod/2, Divide/2
  Divide/1 -> Add/1
  Mod/1 -> Compare To Zero/1
  Cast/1 -> Add/2

== system canBswLib/CanSoftwareVersion/Subsystem1 ==
  state : Inport
  can : Inport  Port=2
  number of messages : Inport  Port=3
  data : Inport  Port=4
  BAM Transfer : Subsystem  TreatAsAtomicUnit=on
  Data Transfer : Subsystem  TreatAsAtomicUnit=on
  Memory : Memory
  String Length : StringLength  OutDataTypeStr=uint8
  wires:
  can/1 -> BAM Transfer/1(can), Data Transfer/1(can)
  String Length/1 -> BAM Transfer/2(message size)
  Memory/1 -> Data Transfer/Trigger
  data/1 -> Data Transfer/3(data), String Length/1
  state/1 -> BAM Transfer/Trigger, Memory/1
  number of messages/1 -> BAM Transfer/3(number of messages), Data Transfer/2(number of messages)

== system canBswLib/СanInit/Function-Call Subsystem ==
  function : TriggerPort  TriggerType=function-call  VariantControl=(inherit)

== system canBswLib/СanInit/Initialize Function ==
  Event Listener : EventListener  DisableCoverage=on  EventName=reset
  bitrate_can_1 : Constant  Value=(bitrate_can_1)  OutDataTypeStr=int32
  bitrate_can_2 : Constant  Value=(bitrate_can_2)  OutDataTypeStr=int32
  bootBrigdeCan1to2 : Constant  Value=bootBrigdeCan1to2Flg  OutDataTypeStr=boolean
  bootBrigdeCan2to1 : Constant  Value=bootBrigdeCan2to1Flg  OutDataTypeStr=boolean
  brigdeCan1to2 : Constant  Value=brigdeCan1to2Flg  OutDataTypeStr=boolean
  brigdeCan2to1 : Constant  Value=brigdeCan2to1Flg  OutDataTypeStr=boolean
  canApi_ConfigBootBridges : can_bswapi/canApi_ConfigBootBridges  SampleTime=-1
  canApi_ConfigBridges : can_bswapi/canApi_ConfigBridges  SampleTime=-1
  canApi_Init : can_bswapi/canApi_Init  SampleTime=-1
  wires:
  brigdeCan2to1/1 -> canApi_ConfigBridges/2
  brigdeCan1to2/1 -> canApi_ConfigBridges/1
  bitrate_can_2/1 -> canApi_Init/2
  bitrate_can_1/1 -> canApi_Init/1
  bootBrigdeCan1to2/1 -> canApi_ConfigBootBridges/1
  bootBrigdeCan2to1/1 -> canApi_ConfigBootBridges/2

== system canBswLib/СanReceiveMsg/CAN Receive ==
  function : TriggerPort  TriggerType=function-call  VariantControl=(inherit)
  can : Constant  Value=(can - 1)  OutDataTypeStr=int32
  canApi_GetMessage : can_bswapi/canApi_GetMessage  SampleTime=-1
  id : Constant  Value=id  OutDataTypeStr=uint32
  msgCnt : Outport
  rxMsg : Outport  Port=2
  wires:
  id/1 -> canApi_GetMessage/2
  can/1 -> canApi_GetMessage/1
  canApi_GetMessage/2 -> rxMsg/1
  canApi_GetMessage/1 -> msgCnt/1

== system canBswLib/СanReceiveMsg/Initialize Function ==
  Event Listener : EventListener  DisableCoverage=on  EventName=reset
  can : Constant  Value=(can - 1)  OutDataTypeStr=int32
  canApi_msgSubscribe : can_bswapi/canApi_msgSubscribe  SampleTime=-1
  id : Constant  Value=id  OutDataTypeStr=uint32
  subscribeStatus : Outport
  wires:
  canApi_msgSubscribe/1 -> subscribeStatus/1
  can/1 -> canApi_msgSubscribe/1
  id/1 -> canApi_msgSubscribe/2

== system canBswLib/СanReceiveMsgTimeout/CAN Receive ==
  function : TriggerPort  TriggerType=function-call  VariantControl=(inherit)
  can : Constant  Value=(can - 1)  OutDataTypeStr=int32
  canGetMessage : can_bswapi/canApi_GetMessage  SampleTime=-1
  id : Constant  Value=id  OutDataTypeStr=uint32
  msgCnt : Outport
  rxMsg : Outport  Port=2
  wires:
  id/1 -> canGetMessage/2
  canGetMessage/1 -> msgCnt/1
  canGetMessage/2 -> rxMsg/1
  can/1 -> canGetMessage/1

== system canBswLib/СanReceiveMsgTimeout/Initialize Function ==
  Event Listener : EventListener  DisableCoverage=on  EventName=reset
  can : Constant  Value=(can - 1)  OutDataTypeStr=int32
  canApi_msgSubscribe : can_bswapi/canApi_msgSubscribe  SampleTime=-1
  id : Constant  Value=id  OutDataTypeStr=uint32
  subscribeStatus : Outport
  wires:
  canApi_msgSubscribe/1 -> subscribeStatus/1
  id/1 -> canApi_msgSubscribe/2
  can/1 -> canApi_msgSubscribe/1

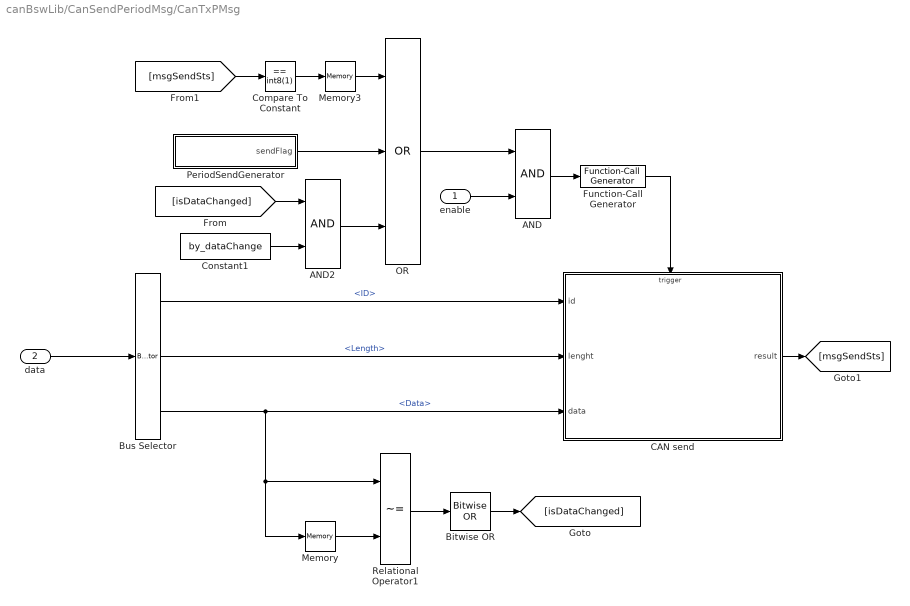
== system canBswLib/СanSendPeriodMsg/CanTxPMsg ==
  enable : Inport  OutDataTypeStr=boolean
  data : Inport  Port=2
  AND : Logic  AllPortsSameDT=off  OutDataTypeStr=boolean
  AND2 : Logic  AllPortsSameDT=off  OutDataTypeStr=boolean
  Bitwise OR : simulink/Logic and Bit Operations/Bitwise Operator  logicop=OR  UseBitMask=off  BitMask=bin2dec('11011001')  BitMaskRealWorld=Stored Integer
      settings: LibrarySourceBlock=|
      | simulink/Quick Insert/Logic and Bit
      | Operations/Bitwise OR
  Bus Selector : BusSelector  OutputSignals=ID,Length,Data
  CAN send : Subsystem  TreatAsAtomicUnit=on
  Compare To Constant : simulink/Logic and Bit Operations/Compare To Constant  relop===  const=int8(1)  OutDataTypeStr=boolean  ZeroCross=off
  Constant1 : Constant  Value=by_dataChange  OutDataTypeStr=boolean
  Function-Call Generator : simulink/Ports & Subsystems/Function-Call Generator  sample_time=sample_time  numberOfIterations=1  DisallowWideOutput=off  ShowEnablePort=on
  Memory : Memory  InheritSampleTime=on
  Memory3 : Memory  InheritSampleTime=on
  OR : Logic  Operator=OR  Inputs=3  AllPortsSameDT=off  OutDataTypeStr=boolean
  PeriodSendGenerator : Subsystem
  Relational Operator1 : RelationalOperator  Operator=~=  OutDataTypeStr=boolean  RndMeth=Simplest  InputSameDT=off
  wires:
  PeriodSendGenerator/1(sendFlag) -> OR/2
  [msgSendSts] -> Compare To Constant/1
  CAN send/1(result) -> [msgSendSts]
  Compare To Constant/1 -> Memory3/1
  [isDataChanged] -> AND2/1
  enable/1 -> AND/2
  AND/1 -> Function-Call Generator/1
  Bitwise OR/1 -> [isDataChanged]
  Constant1/1 -> AND2/2
  Function-Call Generator/1 -> CAN send/Trigger
  Bus Selector/1 -> CAN send/1(id)  "<ID>"
  Memory/1 -> Relational Operator1/2
  Bus Selector/2 -> CAN send/2(lenght)  "<Length>"
  AND2/1 -> OR/3
  Relational Operator1/1 -> Bitwise OR/1
  Bus Selector/3 -> CAN send/3(data), Relational Operator1/1, Memory/1  "<Data>"
  data/1 -> Bus Selector/1
  Memory3/1 -> OR/1
  OR/1 -> AND/1

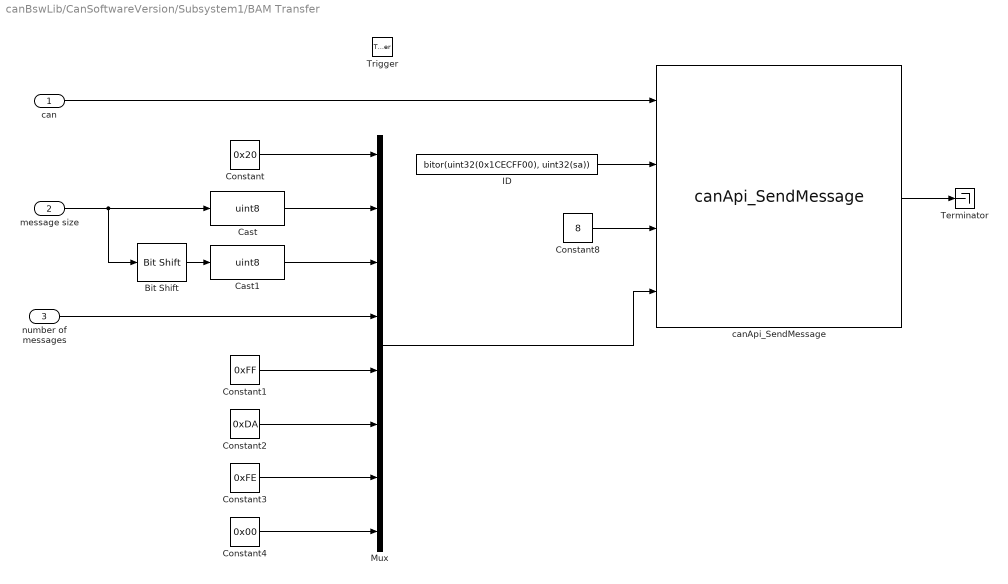
== system canBswLib/CanSoftwareVersion/Subsystem1/BAM Transfer ==
  can : Inport
  message size : Inport  Port=2
  number of messages : Inport  Port=3
  Trigger : TriggerPort  VariantControl=(inherit)
  Bit Shift : hdlsllib/Logic and Bit Operations/Bit Shift  mode=Shift Left Logical  N=8
  Cast : DataTypeConversion  OutDataTypeStr=uint8  RndMeth=Simplest  SaturateOnIntegerOverflow=off
  Cast1 : DataTypeConversion  OutDataTypeStr=uint8  RndMeth=Simplest  SaturateOnIntegerOverflow=off
  Constant : Constant  Value=0x20  OutDataTypeStr=uint8
  Constant1 : Constant  Value=0xFF  OutDataTypeStr=uint8
  Constant2 : Constant  Value=0xDA  OutDataTypeStr=uint8
  Constant3 : Constant  Value=0xFE  OutDataTypeStr=uint8
  Constant4 : Constant  Value=0x00  OutDataTypeStr=uint8
  Constant8 : Constant  Value=8  OutDataTypeStr=uint8
  ID : Constant  Value=bitor(uint32(0x1CECFF00), uint32(sa))  OutDataTypeStr=uint32
  Mux : Mux  Inputs=8
  Terminator : Terminator
  canApi_SendMessage : can_bswapi/canApi_SendMessage  SampleTime=-1
  wires:
  canApi_SendMessage/1 -> Terminator/1
  Mux/1 -> canApi_SendMessage/4
  Constant8/1 -> canApi_SendMessage/3
  ID/1 -> canApi_SendMessage/2
  can/1 -> canApi_SendMessage/1
  Constant4/1 -> Mux/8
  Constant3/1 -> Mux/7
  Constant2/1 -> Mux/6
  Constant1/1 -> Mux/5
  message size/1 -> Cast/1, Bit Shift/1
  Cast/1 -> Mux/2
  Cast1/1 -> Mux/3
  Bit Shift/1 -> Cast1/1
  number of messages/1 -> Mux/4
  Constant/1 -> Mux/1

== system canBswLib/CanSoftwareVersion/Subsystem1/Data Transfer ==
  can : Inport
  number of messages : Inport  Port=2
  data : Inport  Port=3
  Trigger : TriggerPort  VariantControl=(inherit)
  Data transfer : Subsystem  TreatAsAtomicUnit=on
  wires:
  can/1 -> Data transfer/1(can)
  number of messages/1 -> Data transfer/2(number of messages)
  data/1 -> Data transfer/3(data)

== system canBswLib/СanSendPeriodMsg/CanTxPMsg/CAN send ==
  id : Inport
  lenght : Inport  Port=2
  data : Inport  Port=3
  function : TriggerPort  TriggerType=function-call  VariantControl=(inherit)
  can : Constant  Value=(can - 1)  OutDataTypeStr=int32
  canApi_SendMessage : can_bswapi/canApi_SendMessage  SampleTime=-1
  result : Outport
  wires:
  data/1 -> canApi_SendMessage/4
  lenght/1 -> canApi_SendMessage/3
  canApi_SendMessage/1 -> result/1
  id/1 -> canApi_SendMessage/2
  can/1 -> canApi_SendMessage/1

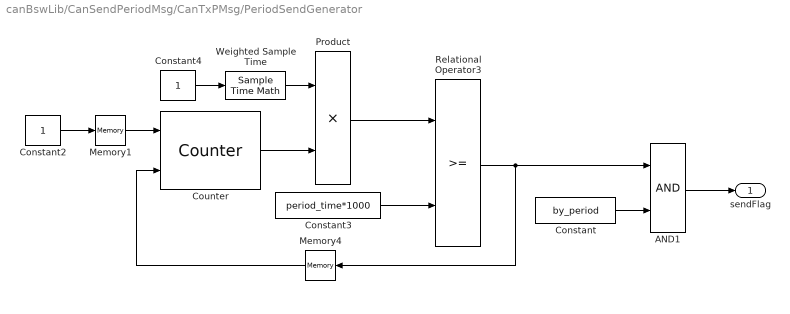
== system canBswLib/СanSendPeriodMsg/CanTxPMsg/PeriodSendGenerator ==
  AND1 : Logic  AllPortsSameDT=off  OutDataTypeStr=boolean
  Constant : Constant  Value=by_period  OutDataTypeStr=boolean
  Constant2 : Constant  OutDataTypeStr=uint32
  Constant3 : Constant  Value=period_time*1000  OutDataTypeStr=uint32
  Constant4 : Constant  OutDataTypeStr=uint32
  Counter : dspswit3/Counter  Direction=Up  CountEvent=Non-zero sample  CounterSize=32 bits  MaxCount=255  InitialCount=0  Output=Count  HitValue=32  ResetInput=on  SamplesPerFrame=1  Ts=-1  CntDtype=uint32  HitDtype=Logical
  Memory1 : Memory  InheritSampleTime=on
  Memory4 : Memory  InheritSampleTime=on
  Product : Product  OutDataTypeStr=uint32  RndMeth=Simplest
  Relational Operator3 : RelationalOperator  OutDataTypeStr=boolean  ZeroCross=off  RndMeth=Simplest  InputSameDT=off
  Weighted Sample Time : SampleTimeMath  TsampMathOp=Ts Only  weightValue=uint32(1000)  OutDataTypeStr=single
  sendFlag : Outport
  wires:
  Constant3/1 -> Relational Operator3/2
  Relational Operator3/1 -> Memory4/1, AND1/1
  Memory1/1 -> Counter/1
  Constant4/1 -> Weighted Sample Time/1
  AND1/1 -> sendFlag/1
  Memory4/1 -> Counter/2
  Constant2/1 -> Memory1/1
  Weighted Sample Time/1 -> Product/1
  Constant/1 -> AND1/2
  Product/1 -> Relational Operator3/1
  Counter/1 -> Product/2

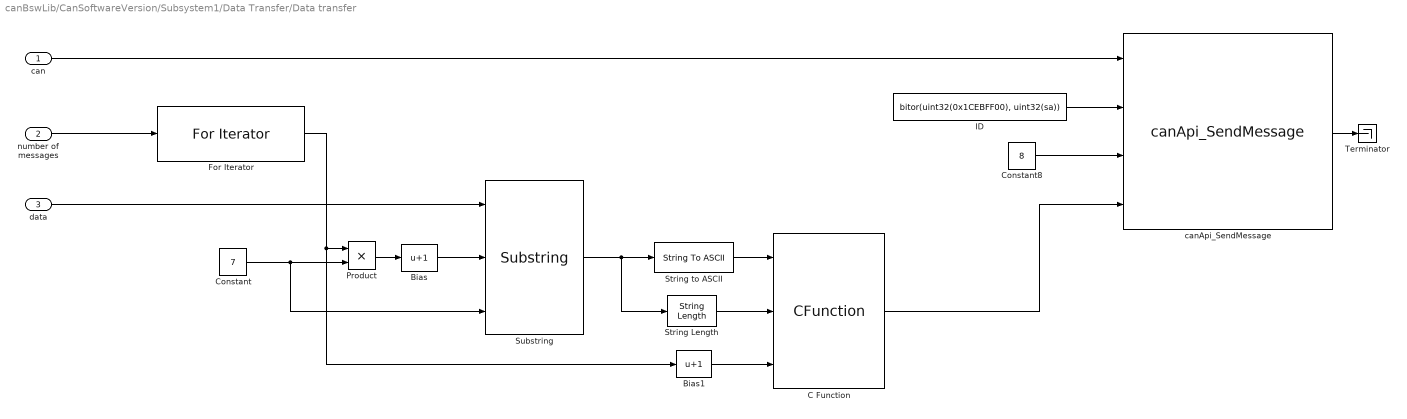
== system canBswLib/CanSoftwareVersion/Subsystem1/Data Transfer/Data transfer ==
  can : Inport
  number of messages : Inport  Port=2
  data : Inport  Port=3
  Bias : Bias  Bias=1  SaturateOnIntegerOverflow=off
  Bias1 : Bias  Bias=1  SaturateOnIntegerOverflow=off
  C Function : CFunction  OutputCode=|
      | if(len < 7)
      | {
      |     data_out[0] = message_number;
      |     for(int i = 0; i < 7; ++i)
      |     {
      |         if(i < len)
      |             data_out[i + 1] = data_in[i];
      |         else
      |             data_out[i + 1] = 0xFF;
      |     }    
      | }
      | else
      | {
      |     data_out[0] = message_number;
      |     for(int i = 0; i < 7; ++i)
      |     {
      |         data_out[i + 1] = data_in[i];    
      |     }   
      | }
  Constant : Constant  Value=7  OutDataTypeStr=uint8
  Constant8 : Constant  Value=8  OutDataTypeStr=uint8
  For Iterator : ForIterator  IterationSource=external  IndexMode=Zero-based  IterationVariableDataType=uint8
  ID : Constant  Value=bitor(uint32(0x1CEBFF00), uint32(sa))  OutDataTypeStr=uint32
  Product : Product  OutDataTypeStr=uint8  RndMeth=Simplest
  String Length : StringLength  OutDataTypeStr=uint32
  String to ASCII : StringToASCII  OutputVectorSize=7
  Substring : Substring
  Terminator : Terminator
  canApi_SendMessage : can_bswapi/canApi_SendMessage  SampleTime=-1
  wires:
  ID/1 -> canApi_SendMessage/2
  Constant8/1 -> canApi_SendMessage/3
  canApi_SendMessage/1 -> Terminator/1
  can/1 -> canApi_SendMessage/1
  C Function/1 -> canApi_SendMessage/4
  String to ASCII/1 -> C Function/1
  Bias1/1 -> C Function/3
  String Length/1 -> C Function/2
  Substring/1 -> String to ASCII/1, String Length/1
  Bias/1 -> Substring/2
  Product/1 -> Bias/1
  For Iterator/1 -> Product/1, Bias1/1
  Constant/1 -> Product/2, Substring/3
  data/1 -> Substring/1
  number of messages/1 -> For Iterator/1
